simulink model "flightControlSystem"  (R2023b)
settings: Solver=ode3  StartTime=0  StopTime=60  FixedStep=Ts  RelTol=1e-3  EnableMultiTasking=on
model workspace (MAT data in the model file):
  deneme_var : Simulink.Parameter (value not decoded)
  gain_1 = 1
  varvar = 5
undefined symbols (not defined in the file): codertarget, Controller, DiscIntNeverNeededParam, Discrete, Estimator, g, gray, init, Sensors, Time, Ts, var_acc_angle_N, var_bias_gyr_N, var_gyro_p_N, Vehicle
libraries: simulink x39, slpidlib x4, ctrlSharedLib x4, sharedtransform x3, parrotlib x1
(part 3 of 3)

== matlab function flightControlSystem/Control System/Path Planning/control1 ==
  data: rel_pointsx input; distx output; rel_pointsy input; disty output
function [distx, disty]= fcn(rel_pointsx, rel_pointsy)
persistent hFig;
persistent hAx;
persistent dom_x;
persistent dom_y;
persistent call_count;
persistent target_chosen;
if isempty(target_chosen)
    target_chosen = 0;
end
distx = 0;
disty = 0;
if isempty(call_count)
    call_count = 0;
end
if isempty(dom_x)
    dom_x = 1;
end
if isempty(dom_y)
    dom_y = -1;
end

% Find the point closest to (0,0)
distances = sqrt(rel_pointsx.^2 + rel_pointsy.^2);
[~, startIndex] = min(distances);
% Pre-allocate sortedPoints to its maximum size
sortedPointsX = zeros(size(rel_pointsx));
sortedPointsY = zeros(size(rel_pointsy));
% Initialize a counter for the next position to fill in sortedPoints
nextIndex = 1;
% Set the first point in sortedPoints
sortedPointsX(nextIndex) = rel_pointsx(startIndex);
sortedPointsY(nextIndex) = rel_pointsy(startIndex);
nextIndex = nextIndex + 1;
used = false(size(rel_pointsx));  % Logical indexing to track used points
used(startIndex) = true;  % Mark the starting point as used
% Now sort the remaining points
while any(~used)
    % Get the last sorted point
    lastPointX = sortedPointsX(nextIndex - 1);
    lastPointY = sortedPointsY(nextIndex - 1);
    % Compute the distances to all remaining points
    distances = sqrt((rel_pointsx(~used) - lastPointX).^2 + (rel_pointsy(~used) - lastPointY).^2);
    % Find the closest point
    [~, idx] = min(distances);
    % Find the original index of the closest point
    originalIdx = find(~used);
    originalIdx = originalIdx(idx);
    % Add the closest point to the sorted points
    sortedPointsX(nextIndex) = rel_pointsx(originalIdx);
    sortedPointsY(nextIndex) = rel_pointsy(originalIdx);
    nextIndex = nextIndex + 1;
    % Mark the closest point as used
    used(originalIdx) = true;
end
rel_pointsx = sortedPointsX;
rel_pointsy = sortedPointsY;
if call_count > 10
    slopes_points = 999*ones(5, 2,20);
    slopes = 999*ones(5);
    slope_counter = 0;
    points_on_a_slope = 1;
    dom = atan2(dom_y, dom_x);
    if_corner = 0;
    last_x = 0;
    last_y = 0;
    corner_x = 0;
    corner_y = 0;
    stop_checking = 0;
    slow_down = 1;
    for i=1:length(rel_pointsx)
        if rel_pointsx(i) ~= 999 && ~stop_checking
            dx = rel_pointsx(i);
            dy = rel_pointsy(i);
            d = sqrt(dx^2+dy^2);
            temp_slope = atan2(dy, dx);
            if abs(dom-temp_slope) < 1.5 && d > 10 && d < 50
                if slope_counter == 0
                    % disp('first slope')
                    slope_counter = slope_counter + 1;
                    slopes(slope_counter) = temp_slope;
                    slopes_points(slope_counter, 1, points_on_a_slope) = rel_pointsx(i);
                    slopes_points(slope_counter, 2, points_on_a_slope) = rel_pointsy(i);
                    dom_x = cos(temp_slope);
                    dom_y = sin(temp_slope);
                    % disp('temp_slope')
                    % disp(temp_slope)
                    last_x = rel_pointsx(i);
                    last_y = rel_pointsy(i);
                elseif abs(temp_slope - slopes(slope_counter))  < 0.2
                    % disp('in the existing slope')
                    points_on_a_slope = points_on_a_slope + 1;
                    slopes_points(slope_counter, 1, points_on_a_slope) = rel_pointsx(i);
                    slopes_points(slope_counter, 2, points_on_a_slope) = rel_pointsy(i);
                    dom_x = cos(temp_slope);
                    dom_y = sin(temp_slope);
                    last_x = rel_pointsx(i);
                    last_y = rel_pointsy(i);
                elseif abs(temp_slope - slopes(slope_counter))  >= 0.2
                    disp('new slope')
                    if_corner = 1;
                    corner_x = rel_pointsx(i);
                    corner_y = rel_pointsy(i);
                    if d > 40
                        disp('d>40')
                        stop_checking = 1;
                    elseif d>10 && d<=40
                        disp('d>10<40')
                        stop_checking = 1;
                        slow_down = 0.3;
                    else
                        disp('<10')
                        slope_counter = slope_counter + 1;
                        slopes(slope_counter) = temp_slope;
                        points_on_a_slope = 1;
                        slopes_points(slope_counter, 1, points_on_a_slope) = rel_pointsx(i);
                        slopes_points(slope_counter, 2, points_on_a_slope) = rel_pointsy(i);
                        dom_x = cos(temp_slope);
                        dom_y = sin(temp_slope);
                        % disp('temp_slope')
                        % disp(temp_slope)
                    end
                end
            end
        end
    end
    if ~if_corner
        distx = cos(atan2(last_y, last_x))*20;
        disty = sin(atan2(last_y, last_x))*20;
    elseif if_corner
        angle_to_corner = atan2(corner_y, corner_x);
        distx = 20*cos(angle_to_corner)*slow_down;
        disty = 20*sin(angle_to_corner)*slow_down;
    end
    disp(slope_counter)
    disp('dom_x')
    disp(dom_x)
    disp('dom_y')
    disp(dom_y)
    if rem(call_count, 30) == 0
        if isempty(hFig)
            % If true, create a new figure and store the handle
            hFig = figure;
            % Create a new axes and store the handle
            hAx = axes('Parent', hFig);
        else
            % If a figure already exists, bring it to the front
            figure(hFig);
        end
        colorss = ['r', 'g', 'b', 'y', 'k'];
        for s = 1:length(slopes)
            if slopes(s) ~= 999
                for p = 1:20
                    if slopes_points(s, 1, p) ~= 999
                        scatter(slopes_points(s, 1, p), slopes_points(s, 2, p), colorss(s))
                        hold on
                    end
                end
            end
        end
        for i=1:length(rel_pointsx)
            if rel_pointsx(i) ~= 999
                scatter(rel_pointsx(i), rel_pointsy(i))
                hold on
            end
        end
        plot([0, 0 + dom_x*100], [0,0 + dom_y*100])
        hold on
        plot([0, 0 + cos(dom + 1.5)*100], [0,0 + sin(dom+ 1.5)*100])
        hold on
        plot([0, 0 + cos(dom-1.5)*100], [0,0 + sin(dom-1.5)*100])
        hold on
        x = 0; y = 0; r = 10;
        hold on
        th = 0:pi/50:2*pi;
        xunit = r * cos(th) + x;
        yunit = r * sin(th) + y;
        plot(xunit, yunit);
        hold on
        r = 50;
        th = 0:pi/50:2*pi;
        xunit = r * cos(th) + x;
        yunit = r * sin(th) + y;
        plot(xunit, yunit);
        axis(hAx, [-60 60 -80 80]);
        hold on
        scatter(0, 0, 'k+', 'filled')
        hold off
        points = rel_pointsx + rel_pointsy;
    end
end
call_count = call_count + 1;
y = 1;
end

== matlab function flightControlSystem/Image Processing System/old_version ==
  data: u input; y output
function y = fcn(u)

% Find contours
image=u;
% Label connected components
[L, num] = bwlabel(image);

% Initialize figure
% figure;
% imshow(image);
% hold on;

% Number of points to plot on each middle line segment
num_points = 5;

% Loop through each connected component to find middle line
for k = 1:num
    % Extract coordinates of the pixels in this component
    [rows, cols] = find(L == k);
    
    % Find the bounding box corners
    min_row = min(rows);
    max_row = max(rows);
    min_col = min(cols);
    max_col = max(cols);
    
    % Compute the centroid
    x_c = (min_col + max_col) / 2;
    y_c = (min_row + max_row) / 2;
    
    % Check the dimensions to decide the orientation
    width = max_col - min_col;
    height = max_row - min_row;
    
    % Initialize variables to hold the start and end coordinates
    x1 = 0; y1 = 0; x2 = 0; y2 = 0;
    
    % If width is greater than height, line is horizontal; else, vertical.
    if width > height
        x1 = min_col;
        y1 = y_c;
        x2 = max_col;
        y2 = y_c;
    else
        x1 = x_c;
        y1 = min_row;
        x2 = x_c;
        y2 = max_row;
    end
    
    % Draw the middle line for this rectangle
    % line([x1, x2], [y1, y2], 'Color', 'r', 'LineWidth', 2);
    
    % Generate points at equal distances along the middle line
    x_points = linspace(x1, x2, num_points);
    y_points = linspace(y1, y2, num_points);
    
    % % Plot these points on the line
    % plot(x_points, y_points, 'go', 'MarkerSize', 6, 'MarkerFaceColor', 'g');
end

% hold off;
y = size(u);

== matlab function flightControlSystem/Control System/Controller/Position Controller/Position error transformation (Earth to Body frame) ==
  data: yaw input; xy_err_earth input; xy_err_body output
function xy_err_body = fcn(yaw,xy_err_earth)

transformation = [cos(yaw), sin(yaw); -sin(yaw),  cos(yaw)];
xy_err_body = transformation * xy_err_earth;


end

== matlab function flightControlSystem/Control System/Path Planning/MATLAB Function ==
  data: pointsx input; y output; pointsy input; dom_x input; dom_y input
function y = fcn(pointsx, pointsy, dom_x, dom_y)

middle_x = 0;
middle_y = 0;

slopes_points = zeros(5, 2,20);
slopes = 99*ones(5);
slopes_counter = 0;
points_on_a_slope = 1;

temp_slope = 0;

for i=1:length(points_x)

    dx = points_x(i);
    dy = points_y(i);
    temp_slope = atan2(dy, dx);


    if slopes_counter == 0 
        
        slope_counter = slope_counter + 1;
        slopes(slope_counter) = temp_slope;
        slopes_points(slope_counter, 1, points_on_a_slope) = points_x(i);
        slopes_points(slope_counter, 2, points_on_a_slope) = points_y(i);

    elseif abs(temp_slope - slopes(slopes_counter))  < 0.09

        points_on_a_slope = points_on_a_slope + 1;
        slopes_points(slope_counter, 1, points_on_a_slope) = points_x(i);
        slopes_points(slope_counter, 2, points_on_a_slope) = points_y(i);

    elseif abs(temp_slope - slopes(slopes_counter))  >= 0.09

        slope_counter = slope_counter + 1;
        slopes(slope_counter) = temp_slope;
        points_on_a_slope = 1;
        slopes_points(slope_counter, 1, points_on_a_slope) = points_x(i);
        slopes_points(slope_counter, 2, points_on_a_slope) = points_y(i);

        
    end


end

%Find the closest po

% persistent hFig;
% persistent hAx;
% 
% if isempty(hFig)
%     % If true, create a new figure and store the handle
%     hFig = figure;
%     % Create a new axes and store the handle
%     hAx = axes('Parent', hFig);
% else
%     % If a figure already exists, bring it to the front
%     figure(hFig);
% end
% scatter(pointsx, pointsy)
% axis(hAx, [-60 60 -80 80]);



points = pointsx + pointsy;

y = points;

end

== matlab function flightControlSystem/Image Processing System/new_version ==
  data: u input; outt output; distX output; distY output; pointsx output; pointsy output
function [outt, distX, distY, pointsx, pointsy] = fcn(u)
persistent call_count;
persistent hFig;
persistent hAx;
persistent rmse_lin;

rmse_lin = 9999*ones(1000);

if isempty(call_count)
    call_count = 1;
end

% Clean up the binary image using morphological operations
cleanedImage = bwmorph(u, 'clean');

% Thinning the image to get the centerline
centerline = bwmorph(cleanedImage, 'thin', Inf);

% Removing spurs iteratively
numIterationsToRemoveSpurs = 15;  % Adjust this based on the branch lengths you want to remove
for k = 1:numIterationsToRemoveSpurs
    centerline = bwmorph(centerline, 'spur');
end

% Creating an RGB image
redChannel = cleanedImage & ~centerline;
greenChannel = cleanedImage & ~centerline;
blueChannel = cleanedImage & ~centerline;

outt = uint8(cat(3, redChannel, greenChannel, blueChannel) * 255);

[yIdx, xIdx] = find(centerline);

% Pre-allocate maximum size for filtered points
filteredX = zeros(size(xIdx));
filteredY = zeros(size(yIdx));
count = 0;

for i = 1:length(xIdx)
    if count == 0
        count = count + 1;
        filteredX(count) = xIdx(i);
        filteredY(count) = yIdx(i);
    else
        minDistances = sqrt((filteredX(1:count) - xIdx(i)).^2 + (filteredY(1:count) - yIdx(i)).^2);
        if all(minDistances > 10)
            count = count + 1;
            filteredX(count) = xIdx(i);
            filteredY(count) = yIdx(i);
        end
    end
end

% Truncate arrays to the number of filtered points
filteredX = filteredX(1:count);
filteredY = filteredY(1:count);

% disp("Filtered xs are:");
% disp(filteredX);
% disp("Filtered ys are:");
% disp(filteredY);
% disp("all");

% Find the middle point of the image
middleX = size(u, 2) / 2;
middleY = size(u, 1) / 2;

% Translate the coordinates so that the middle point becomes (0,0)
filteredX = filteredX - middleX;
filteredY = filteredY - middleY;

% Compute distances from each point in the filtered list to the middle point
distancesToMiddle = sqrt((filteredX - middleX).^2 + (filteredY - middleY).^2);

% Sort the distances and get indices of the 20 smallest distances
[~, sortedIndices] = sort(distancesToMiddle, 'ascend');
closestIndices = sortedIndices(1:min(20, length(sortedIndices)));

% Assign points_x and points_y to the x and y coordinates of the 20 closest points from the filtered list
pointsx = 999 * ones(20, 1);
pointsy = 999 * ones(20, 1);

pointsx(1:length(closestIndices)) = filteredX(closestIndices);
pointsy(1:length(closestIndices)) = filteredY(closestIndices);

% Remove points with coordinates (999,999)
validPoints = pointsx ~= 999 & pointsy ~= 999;
unsorted_validX = pointsx(validPoints);
unsorted_validY = pointsy(validPoints);
flip_flag = 0;

if length(unsorted_validX) >= 3 && all(isfinite(unsorted_validX))
    % Ensure x-values are finite and sort data if necessary
    % Sort data while keeping the corresponding y-values aligned

    for i = 1:length(unsorted_validX)
        unsorted_validX(i) = unsorted_validX(i) + randn * 1.5;
        unsorted_validY(i) = unsorted_validY(i) + randn * 1.5;
    end

    % if std(validX) < 10
    %     flip_flag = 1;
    %     temp = validY;
    %     validY = validX;
    %     validX = temp;
    % end

    [validX, sortIdx] = sort(unsorted_validX);
    validY = unsorted_validY(sortIdx);

    % Fit a second order polynomial to the valid points
    p = polyfit(validX, validY, 2);
    % pp = pchip(validX, validY);
        disp("start")
    % disp(pp)
    disp(validX)
    %  disp(std(validX))
     disp("finish")
    % % disp("p1")
    % % disp(p(1))
    % % disp("p2")
    % % disp(p(2))
    % % disp("p3")
    % % disp(p(3))
    % % The coefficients p(1), p(2), and p(3) correspond to the quadratic, linear, and constant terms of the polynomial, respectively.
    % 
    % % If you want to visualize the curve on your image, you can generate y values for a range of x values using the polyval function.
    % xValues = min(validX):0.1:max(validX);  % Adjust the step size as needed for your image resolution
    % yValues = ppval(pp, xValues);

    % xValues = min(validX):0.1:max(validX);  % Adjust the step size as needed for your image resolution
    numPoints = 200;  % Calculate the number of points

    xvaluesi = linspace(1, numel(validX), numPoints);  % New x-vector with 20 elements
    xValues = interp1(1:numel(validX), validX, xvaluesi, 'pchip');  % Interpolate to new x-vector
    disp(xValues)

    % xValues = linspace(min(validX), max(validX), numPoints);  % Generate linearly spaced vector
    % yValues = ppval(pp, xValues);
    % yValues = sgolayfilt(yValues,3,19);
    yValues = polyval(p, xValues);
    % valid_y_for_rmse = polyval(p, validX);
    % RMSE_linear = sqrt(mean(validY-valid_y_for_rmse).^2);
    % rmse_lin(call_count) = RMSE_linear;
    % assignin('base', 'rmse_lin', 'rmse_lin_output');
    % yValues = interp1(validX, validY, xValues, 'linear', 'extrap');

        % Check if the figure handle is empty or the figure is closed
    if isempty(hFig) 
        % If true, create a new figure and store the handle
        hFig = figure;
        % Create a new axes and store the handle
        hAx = axes('Parent', hFig);        
    else
        % If a figure already exists, bring it to the front
        figure(hFig);
    end

    plot(hAx, xValues, yValues);
    hold on
    scatter(validX, validY)
    hold off
    axis(hAx, [-60 60 -80 80]);


    if flip_flag == 1
        % Convert the x and y values back to the original coordinate system for plotting
        xValues = yValues + middleY;
        yValues = xValues + middleX;
    else
        % Convert the x and y values back to the original coordinate system for plotting
        xValues = xValues + middleX;
        yValues = yValues + middleY;
    end
    
    % Now you can use these xValues and yValues to draw the curve on your image
    for i = 1:length(xValues)
        x = round(xValues(i));
        y = round(yValues(i));
        if x > 0 && x <= size(outt, 2) && y > 0 && y <= size(outt, 1)
            outt(y, x, 1) = 0;   % Red channel
            outt(y, x, 2) = 0;     % Green channel
            outt(y, x, 3) = 255;     % Blue channel
        end
    end
end

% Drawing green circles manually
radius = 4;
for k = 1:length(filteredX)
    for dx = -radius:radius
        for dy = -radius:radius
            if dx^2 + dy^2 <= radius^2
                x = filteredX(k) + dx + middleX;  % Add middleX
                y = filteredY(k) + dy + middleY;  % Add middleY
                if x > 0 && x <= size(outt, 2) && y > 0 && y <= size(outt, 1)
                    outt(y, x, 1) = 0;     % Red channel
                    outt(y, x, 2) = floor(255*k/length(filteredX));   % Green channel
                    outt(y, x, 3) = 0;     % Blue channel
                end
            end
        end
    end
end

if call_count < 75
    distX=-10;
    distY=0;
elseif call_count >= 60 && call_count<120
    distX=0;
    distY=30;
else
    distX=0;
    distY=0;
end

call_count = call_count + 1;

end

== matlab function flightControlSystem/Image Processing System/send_only_points1 ==
  data: u input; outt output; distX output; distY output; dom_x output; dom_y output; pointsx output; pointsy output
function [outt, distX, distY, dom_x, dom_y, pointsx, pointsy] = fcn(u)
persistent call_count;
% persistent hFig;
% persistent hAx;

if isempty(call_count)
    call_count = 1;
end

% Clean up the binary image using morphological operations
cleanedImage = bwmorph(u, 'clean');

% se = strel('disk', 1);
% 
% eroded_image = imerode(cleanedImage, se);
% 
% boundaries = cleanedImage - eroded_image;
% 
% boundaries = imbinarize(boundaries);
% 
cleanedImage = imgaussfilt(im2uint8(cleanedImage),4);

% Thinning the image to get the centerline
centerline = bwmorph(cleanedImage, 'thin', Inf);

centerline = bwmorph(centerline, 'spur', 20);

% Creating an RGB image
redChannel = cleanedImage & ~centerline;
greenChannel = cleanedImage & ~centerline;
blueChannel = cleanedImage & ~centerline;

outt = uint8(cat(3, redChannel, greenChannel, blueChannel) * 255);

[yIdx, xIdx] = find(centerline);

% Pre-allocate maximum size for filtered points
filteredX = zeros(size(xIdx));
filteredY = zeros(size(yIdx));
count = 0;

for i = 1:length(xIdx)
    if count == 0
        count = count + 1;
        filteredX(count) = xIdx(i);
        filteredY(count) = yIdx(i);
    else
        minDistances = sqrt((filteredX(1:count) - xIdx(i)).^2 + (filteredY(1:count) - yIdx(i)).^2);
        if all(minDistances > 7)
            count = count + 1;
            filteredX(count) = xIdx(i);
            filteredY(count) = yIdx(i);
        end
    end
end

% Truncate arrays to the number of filtered points
filteredX = filteredX(1:count);
filteredY = filteredY(1:count);

% disp("Filtered xs are:");
% disp(filteredX);
% disp("Filtered ys are:");
% disp(filteredY);
% disp("all");

% Find the middle point of the image
middleX = size(u, 2) / 2;
middleY = size(u, 1) / 2;

% Translate the coordinates so that the middle point becomes (0,0)
filteredX = filteredX - middleX;
filteredY = filteredY - middleY;

% Compute distances from each point in the filtered list to the middle point
distancesToMiddle = sqrt((filteredX - middleX).^2 + (filteredY - middleY).^2);

% Sort the distances and get indices of the 20 smallest distances
N_points = 40;

[~, sortedIndices] = sort(distancesToMiddle, 'ascend');
closestIndices = sortedIndices(1:min(N_points, length(sortedIndices)));

% Assign points_x and points_y to the x and y coordinates of the 20 closest points from the filtered list
pointsx = 999 * ones(N_points, 1);
pointsy = 999 * ones(N_points, 1);

pointsx(1:length(closestIndices)) = filteredX(closestIndices);
pointsy(1:length(closestIndices)) = filteredY(closestIndices);

% Remove points with coordinates (999,999)
validPoints = pointsx ~= 999 & pointsy ~= 999;
unsorted_validX = pointsx(validPoints);
unsorted_validY = pointsy(validPoints);

if length(unsorted_validX) >= 3 && all(isfinite(unsorted_validX))
    % Ensure x-values are finite and sort data if necessary
    % Sort data while keeping the corresponding y-values aligned

    [validX, sortIdx] = sort(unsorted_validX);
    validY = unsorted_validY(sortIdx);


    %     % Check if the figure handle is empty or the figure is closed
    % if isempty(hFig) 
    %     % If true, create a new figure and store the handle
    %     hFig = figure;
    %     % Create a new axes and store the handle
    %     hAx = axes('Parent', hFig);        
    % else
    %     % If a figure already exists, bring it to the front
    %     figure(hFig);
    % end
    % 
    % scatter(validX, validY)
    % axis(hAx, [-60 60 -80 80]);

end

% Drawing green circles manually
radius = 4;
for k = 1:length(filteredX)
    for dx = -radius:radius
        for dy = -radius:radius
            if dx^2 + dy^2 <= radius^2
                x = filteredX(k) + dx + middleX;  % Add middleX
                y = filteredY(k) + dy + middleY;  % Add middleY
                if x > 0 && x <= size(outt, 2) && y > 0 && y <= size(outt, 1)
                    outt(y, x, 1) = 0;     % Red channel
                    outt(y, x, 2) = floor(255*k/length(filteredX));   % Green channel
                    outt(y, x, 3) = 0;     % Blue channel
                end
            end
        end
    end
end

    for dx = -radius:radius
        for dy = -radius:radius
            if dx^2 + dy^2 <= radius^2
                x = middleX;  % Add middleX
                y = middleY;  % Add middleY
                if x > 0 && x <= size(outt, 2) && y > 0 && y <= size(outt, 1)
                    outt(y, x, 1) = 255;     % Red channel
                    outt(y, x, 2) = 0;   % Green channel
                    outt(y, x, 3) = 0;     % Blue channel
                end
            end
        end
    end

% distX=0;
% distY=30;

if call_count < 55
    distX=0;
    distY=20;
    dom_x = 0;
    dom_y = 1;
elseif call_count >= 60 && call_count<100
    distX=20;
    distY=0;
    dom_x = -1;
    dom_y = 0;
else
    dom_x = 0;
    dom_y = 0;
    distX=0;
    distY=0;
end

call_count = call_count + 1;

end

== matlab function flightControlSystem/Image Processing System/tugay_deneme1 ==
  data: u input; outt output; distX output; distY output; pointsx output; pointsy output
function [outt, distX, distY, pointsx, pointsy] = fcn(u)
persistent call_count;
persistent hFig;
persistent hAx;

if isempty(call_count)
    call_count = 1;
end

% Clean up the binary image using morphological operations
cleanedImage = bwmorph(u, 'clean');

% Thinning the image to get the centerline
centerline = bwmorph(cleanedImage, 'thin', Inf);

% Removing spurs iteratively
numIterationsToRemoveSpurs = 15;  % Adjust this based on the branch lengths you want to remove
for k = 1:numIterationsToRemoveSpurs
    centerline = bwmorph(centerline, 'spur');
end

% Creating an RGB image
redChannel = cleanedImage & ~centerline;
greenChannel = cleanedImage & ~centerline;
blueChannel = cleanedImage & ~centerline;

outt = uint8(cat(3, redChannel, greenChannel, blueChannel) * 255);

[yIdx, xIdx] = find(centerline);

% Pre-allocate maximum size for filtered points
filteredX = zeros(size(xIdx));
filteredY = zeros(size(yIdx));
count = 0;

for i = 1:length(xIdx)
    if count == 0
        count = count + 1;
        filteredX(count) = xIdx(i);
        filteredY(count) = yIdx(i);
    else
        minDistances = sqrt((filteredX(1:count) - xIdx(i)).^2 + (filteredY(1:count) - yIdx(i)).^2);
        if all(minDistances > 10)
            count = count + 1;
            filteredX(count) = xIdx(i);
            filteredY(count) = yIdx(i);
        end
    end
end

% Truncate arrays to the number of filtered points
filteredX = filteredX(1:count);
filteredY = filteredY(1:count);

% disp("Filtered xs are:");
% disp(filteredX);
% disp("Filtered ys are:");
% disp(filteredY);
% disp("all");

% Find the middle point of the image
middleX = size(u, 2) / 2;
middleY = size(u, 1) / 2;

% Translate the coordinates so that the middle point becomes (0,0)
filteredX = filteredX - middleX;
filteredY = filteredY - middleY;

% Initialize sorted points with a size of 20, filled with value 999
sortedPointsX = 999 * ones(20, 1);
sortedPointsY = 999 * ones(20, 1);
sorted_count = 1;  % starting at 1 as the middle point is the first point

% Assign the middle point to the first position
sortedPointsX(1) = middleX;
sortedPointsY(1) = middleY;

while ~isempty(filteredX) && sorted_count < 20
    % Compute distances from the last sorted point to all unsorted points
    distances = sqrt((sortedPointsX(sorted_count) - filteredX).^2 + (sortedPointsY(sorted_count) - filteredY).^2);
    
    % Find the index of the closest point
    [~, closestIdx] = min(distances);
    
    % Increment the count
    sorted_count = sorted_count + 1;
    
    % Add the closest point to the sorted list
    sortedPointsX(sorted_count) = filteredX(closestIdx);
    sortedPointsY(sorted_count) = filteredY(closestIdx);
    
    % Remove the closest point from the list of points to be sorted
    filteredX(closestIdx) = [];
    filteredY(closestIdx) = [];
end

% % Assign points_x and points_y to the x and y coordinates of the 20 closest points from the filtered list
% pointsx = 999 * ones(20, 1);
% pointsy = 999 * ones(20, 1);

% Assign points_x and points_y to the x and y coordinates of the 20 closest points from the sorted list
pointsx = sortedPointsX;
pointsy = sortedPointsY;

% Remove points with coordinates (999,999)
validPoints = pointsx ~= 999 & pointsy ~= 999;
unsorted_validX = pointsx(validPoints);
unsorted_validY = pointsy(validPoints);

if length(unsorted_validX) >= 3 && all(isfinite(unsorted_validX))
    % Ensure x-values are finite and sort data if necessary
    % Sort data while keeping the corresponding y-values aligned

    % [validX, sortIdx] = sort(unsorted_validX);
    % validY = unsorted_validY(sortIdx);


        % Check if the figure handle is empty or the figure is closed
    if isempty(hFig) 
        % If true, create a new figure and store the handle
        hFig = figure;
        % Create a new axes and store the handle
        hAx = axes('Parent', hFig);        
    else
        % If a figure already exists, bring it to the front
        figure(hFig);
    end

    scatter(pointsx, pointsy)
    axis(hAx, [-60 60 -80 80]);
    labels = ['1', '2', '3', '4', '5', '6', '7', '8', '9', "10", "11", "12", "13", "14", "15", "16", "17", "18", "19", "20"];

    for i = 1:length(pointsx)
        text(pointsx(i), pointsy(i), labels(i), 'HorizontalAlignment', 'left', 'VerticalAlignment', 'top');
    end

end

% Drawing green circles manually
radius = 4;
for k = 2:length(sortedPointsX)
    for dx = -radius:radius
        for dy = -radius:radius
            if dx^2 + dy^2 <= radius^2
                x = sortedPointsX(k) + dx + middleX;  % Add middleX
                y = sortedPointsY(k) + dy + middleY;  % Add middleY
                if x > 0 && x <= size(outt, 2) && y > 0 && y <= size(outt, 1)
                    outt(y, x, 1) = 0;     % Red channel
                    outt(y, x, 2) = floor(255*k/length(sortedPointsX));   % Green channel
                    outt(y, x, 3) = 0;     % Blue channel
                end
            end
        end
    end
end

if call_count < 75
    distX=-10;
    distY=10;
elseif call_count >= 60 && call_count<120
    distX=10;
    distY=10;
else
    distX=0;
    distY=0;
end

call_count = call_count + 1;

end

== matlab function flightControlSystem/Image Processing System/sloper ==
  data: pointsx input; distx output; pointsy input; disty output
function [distx, disty]= fcn(pointsx, pointsy)

persistent hFig;
persistent hAx;
persistent dom;
persistent call_count;
persistent if_corner;

distx = 0;
disty = 0;

if isempty(dom)
    dom = deg2rad(90);
end

if isempty(if_corner)
    if_corner = 0;
end

if isempty(call_count)
call_count = 0;
end

pointsy = -pointsy;

% Find the point closest to (0,0)
distances = sqrt(pointsx.^2 + pointsy.^2);
[~, startIndex] = min(distances);
% Pre-allocate sortedPoints to its maximum size
sortedPointsX = zeros(size(pointsx));
sortedPointsY = zeros(size(pointsy));
% Initialize a counter for the next position to fill in sortedPoints
nextIndex = 1;
% Set the first point in sortedPoints
sortedPointsX(nextIndex) = pointsx(startIndex);
sortedPointsY(nextIndex) = pointsy(startIndex);
nextIndex = nextIndex + 1;
used = false(size(pointsx)); % Logical indexing to track used points
used(startIndex) = true; % Mark the starting point as used
% Now sort the remaining points
while any(~used)
    % Get the last sorted point
    lastPointX = sortedPointsX(nextIndex - 1);
    lastPointY = sortedPointsY(nextIndex - 1);
    % Compute the distances to all remaining points
    distances = sqrt((pointsx(~used) - lastPointX).^2 + (pointsy(~used) - lastPointY).^2);
    % Find the closest point
    [~, idx] = min(distances);
    % Find the original index of the closest point
    originalIdx = find(~used);
    originalIdx = originalIdx(idx);
    % Add the closest point to the sorted points
    sortedPointsX(nextIndex) = pointsx(originalIdx);
    sortedPointsY(nextIndex) = pointsy(originalIdx);
    nextIndex = nextIndex + 1;
    % Mark the closest point as used
    used(originalIdx) = true;
end
pointsx = sortedPointsX;
pointsy = sortedPointsY;

if call_count > 10

        slope = 999;
        ac_slope = 999;
        temp_slope = 0;
        last_x = 0;
        last_y = 0;
        corner_x = 0;
        corner_y = 0;
        stop_checking = 0;
        slow_down = 1;

        for i=1:length(pointsx)

            if pointsx(i) ~= 999

                dx = pointsx(i);
                dy = pointsy(i);
                d = sqrt(dx^2+dy^2);
                temp_slope = atan2(dy, dx);

                if abs(dom-temp_slope) < 1.5 && d > 10 && d < 50

                    if slope == 999

                        slope = temp_slope;
                        last_x = pointsx(i);
                        last_y = pointsy(i);
                        dom = atan2(last_y, last_x);

                    elseif abs(temp_slope - slope) < 0.2

                        last_x = pointsx(i);
                        last_y = pointsy(i);

                    elseif abs(temp_slope - slopes(slope_counter)) >= 0.2

                        if ~if_corner
                            
                            corner_x = pointsx(i);
                            corner_y = pointsy(i);
                            if_corner = 1;

                            if d > 40 
    
                                last_x = pointsx(i);
                                last_y = pointsy(i); 
                                dom = atan2(last_y, last_x);
    
                            elseif d>10 && d<=40 
    
                                last_x = pointsx(i);
                                last_y = pointsy(i); 
                                slow_down = 0.3;
                                dom = atan2(last_y, last_x);
    
                            else
                                
                                if_corner = 0;
    
                            end


                        end
                  

                    end

                end




            end



        end



    


end



end

== matlab function flightControlSystem/Image Processing System/sloper_old ==
  data: pointsx input; distx output; pointsy input; disty output
function [distx, disty]= fcn(pointsx, pointsy)

persistent hFig;
persistent hAx;
persistent dom_x;
persistent dom_y;
persistent call_count;
persistent target_chosen;

if isempty(target_chosen)
    target_chosen = 0;
end

distx = 0;
disty = 0;

if isempty(call_count)
    call_count = 0;
end

if isempty(dom_x)
    dom_x = 1;
end

if isempty(dom_y)
    dom_y = -1;
end

pointsy = -pointsy;

% offset_x, offset_y = heading_proj(curr_state)

% Find the point closest to (0,0)
distances = sqrt(pointsx.^2 + pointsy.^2);
[~, startIndex] = min(distances);

% Pre-allocate sortedPoints to its maximum size
sortedPointsX = zeros(size(pointsx));
sortedPointsY = zeros(size(pointsy));
% Initialize a counter for the next position to fill in sortedPoints
nextIndex = 1;
% Set the first point in sortedPoints
sortedPointsX(nextIndex) = pointsx(startIndex);
sortedPointsY(nextIndex) = pointsy(startIndex);
nextIndex = nextIndex + 1;
used = false(size(pointsx));  % Logical indexing to track used points
used(startIndex) = true;  % Mark the starting point as used

% Now sort the remaining points
while any(~used)
    % Get the last sorted point
    lastPointX = sortedPointsX(nextIndex - 1);
    lastPointY = sortedPointsY(nextIndex - 1);
    % Compute the distances to all remaining points
    distances = sqrt((pointsx(~used) - lastPointX).^2 + (pointsy(~used) - lastPointY).^2);
    % Find the closest point
    [~, idx] = min(distances);
    % Find the original index of the closest point
    originalIdx = find(~used);
    originalIdx = originalIdx(idx);
    % Add the closest point to the sorted points
    sortedPointsX(nextIndex) = pointsx(originalIdx);
    sortedPointsY(nextIndex) = pointsy(originalIdx);
    nextIndex = nextIndex + 1;
    % Mark the closest point as used
    used(originalIdx) = true;
end

pointsx = sortedPointsX;
pointsy = sortedPointsY;

if call_count > 10

    slopes_points = 999*ones(5, 2,20);
    slopes = 999*ones(5);
    slope_counter = 0;
    points_on_a_slope = 1;

    dom = atan2(dom_y, dom_x);
    if_corner = 0;
    last_x = 0;
    last_y = 0;
    corner_x = 0;
    corner_y = 0;
    stop_checking = 0;
    slow_down = 1;


    for i=1:length(pointsx)

        if pointsx(i) ~= 999 && ~stop_checking

            dx = pointsx(i);
            dy = pointsy(i);
            d = sqrt(dx^2+dy^2);
            temp_slope = atan2(dy, dx);

            if abs(dom-temp_slope) < 1.5 && d > 10 && d < 50 

                if slope_counter == 0
                    % disp("first slope")
                    slope_counter = slope_counter + 1;
                    slopes(slope_counter) = temp_slope;
                    slopes_points(slope_counter, 1, points_on_a_slope) = pointsx(i);
                    slopes_points(slope_counter, 2, points_on_a_slope) = pointsy(i);
                    dom_x = cos(temp_slope);
                    dom_y = sin(temp_slope);
                    % disp("temp_slope")
                    % disp(temp_slope)
                    last_x = pointsx(i);
                    last_y = pointsy(i);                    

                elseif abs(temp_slope - slopes(slope_counter))  < 0.2
                    % disp("in the existing slope")
                    points_on_a_slope = points_on_a_slope + 1;
                    slopes_points(slope_counter, 1, points_on_a_slope) = pointsx(i);
                    slopes_points(slope_counter, 2, points_on_a_slope) = pointsy(i);
                    dom_x = cos(temp_slope);
                    dom_y = sin(temp_slope);
                    last_x = pointsx(i);
                    last_y = pointsy(i);

                elseif abs(temp_slope - slopes(slope_counter))  >= 0.2
                    disp("new slope")
                    if_corner = 1;
                    corner_x = pointsx(i);
                    corner_y = pointsy(i);

                    if d > 40
                        disp("d>40")
                        stop_checking = 1;
                    elseif d>10 && d<=40
                        disp("d>10<40")
                        stop_checking = 1;
                        slow_down = 0.3;
                    else
                        disp("<10")
                        slope_counter = slope_counter + 1;
                        slopes(slope_counter) = temp_slope;
                        points_on_a_slope = 1;
                        slopes_points(slope_counter, 1, points_on_a_slope) = pointsx(i);
                        slopes_points(slope_counter, 2, points_on_a_slope) = pointsy(i);
                        dom_x = cos(temp_slope);
                        dom_y = sin(temp_slope);
                        % disp("temp_slope")
                        % disp(temp_slope)
                    end


                end

            end
        end
    end

    if ~if_corner
        
        distx = cos(atan2(last_y, last_x))*20;
        disty = sin(atan2(last_y, last_x))*20;

    elseif if_corner 

        angle_to_corner = atan2(corner_y, corner_x);
        distx = 20*cos(angle_to_corner)*slow_down;
        disty = 20*sin(angle_to_corner)*slow_down;

    end

    % disp(slope_counter)

    % disp("dom_x")
    % disp(dom_x)
    % disp("dom_y")
    % disp(dom_y)

    if isempty(hFig)
        % If true, create a new figure and store the handle
        hFig = figure;
        % Create a new axes and store the handle
        hAx = axes('Parent', hFig);
    else
        % If a figure already exists, bring it to the front
        figure(hFig);
    end

    colorss = ['r', 'g', 'b', 'y', 'k'];

    for s = 1:length(slopes)
        if slopes(s) ~= 999
            for p = 1:20
                if slopes_points(s, 1, p) ~= 999
                    scatter(slopes_points(s, 1, p), slopes_points(s, 2, p), colorss(s))
                    hold on
                end
            end
        end
    end



    % for i=1:length(pointsx)
    %     if pointsx(i) ~= 999
    %         scatter(pointsx(i), pointsy(i))
    %         hold on
    %     end
    % end

    plot([0, 0 + dom_x*100], [0,0 + dom_y*100])
    hold on
    plot([0, 0 + cos(dom + 1.5)*100], [0,0 + sin(dom+ 1.5)*100])
    hold on
    plot([0, 0 + cos(dom-1.5)*100], [0,0 + sin(dom-1.5)*100])
    hold on
    x = 0; y = 0; r = 10;
    hold on
    th = 0:pi/50:2*pi;
    xunit = r * cos(th) + x;
    yunit = r * sin(th) + y;
    plot(xunit, yunit);
    hold on
    r = 50;
    th = 0:pi/50:2*pi;
    xunit = r * cos(th) + x;
    yunit = r * sin(th) + y;
    plot(xunit, yunit);
    axis(hAx, [-60 60 -80 80]);
    hold off



    points = pointsx + pointsy;



end
call_count = call_count + 1;
y = 1;
end

== matlab function flightControlSystem/Control System/Path Planning/cam2rel ==
  data: pointsx input; rel_pointsx output; pointsy input; rel_pointsy output; pitch input; roll input
function [rel_pointsx, rel_pointsy]= cam2rel(pointsx, pointsy, pitch, roll)
persistent call_count;
if isempty(call_count)
    call_count = 0;
end

fov_x = 32;
fov_y = 32;
img_w = 160;
img_h = 120;
offset_y = -tan(pitch)/tan(fov_y/2)*0.5*img_h;
offset_x = -tan(-roll)/tan(fov_x/2)*0.5*img_w;

rel_pointsx = pointsx + offset_x;
rel_pointsy = -pointsy + offset_y;

call_count = call_count+1;
end
